simulink model "inverted_pendulum_simulink"  (R2023a)
settings: Solver=VariableStepAuto  StartTime=0.0  StopTime=10  RelTol=1e-3
values from neighbouring files (symbols this model uses):
  A = double(A)    [Inverted_pendulum_compute.m]
  B = double(B)    [Inverted_pendulum_compute.m]
  K = lqr(sys, Q, R)    [Inverted_pendulum_compute.m]
settings Model: Creator=belov  LastModifiedBy=belov

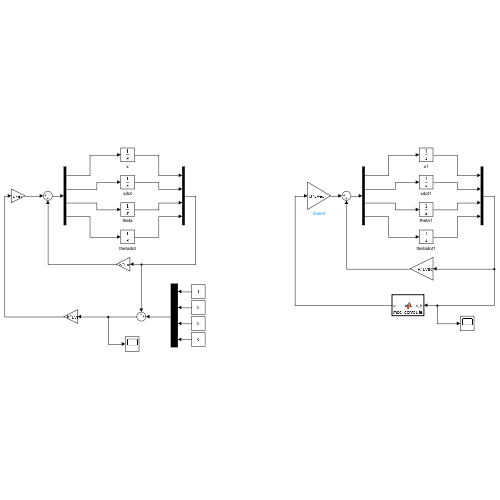
[thumbnail: Simulink's stored preview of the top-level diagram]
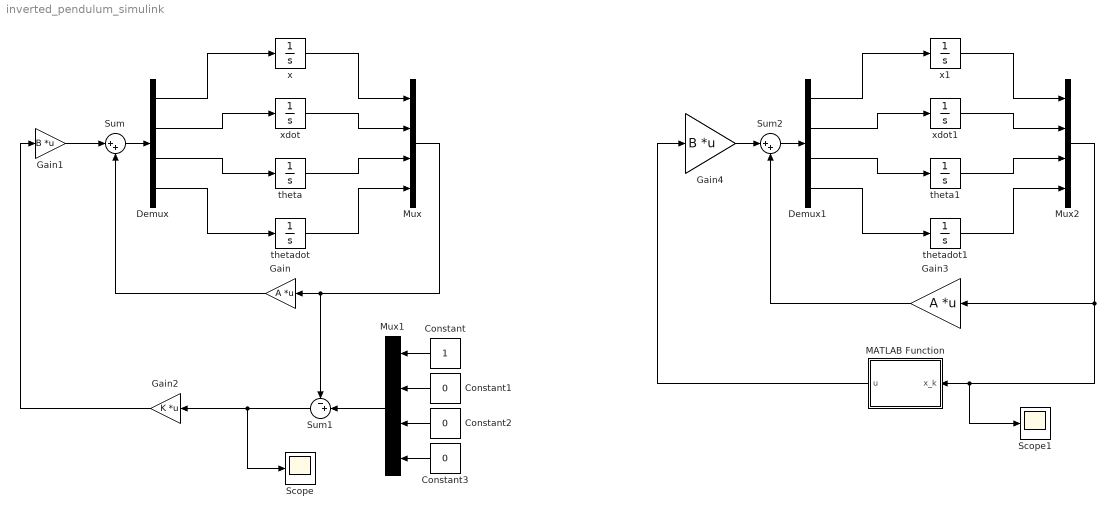
== system inverted_pendulum_simulink ==
  Constant : Constant
  Constant1 : Constant  Value=0
  Constant2 : Constant  Value=0
  Constant3 : Constant  Value=0
  Demux : Demux
  Demux1 : Demux
  Gain : Gain  Gain=A  Multiplication=Matrix(K*u) (u vector)
  Gain1 : Gain  Gain=B  Multiplication=Matrix(K*u) (u vector)
  Gain2 : Gain  Gain=K  Multiplication=Matrix(K*u) (u vector)
  Gain3 : Gain  Gain=A  Multiplication=Matrix(K*u) (u vector)
  Gain4 : Gain  Gain=B  Multiplication=Matrix(K*u) (u vector)
  MATLAB Function : MATLAB Function  TreatAsAtomicUnit=on  SystemSampleTime=0.01
  Mux : Mux
  Mux1 : Mux
  Mux2 : Mux
  Scope : Scope
  Scope1 : Scope
  Sum : Sum  Inputs=|++
  Sum1 : Sum  Inputs=-+|
  Sum2 : Sum  Inputs=|++
  theta : Integrator
  theta1 : Integrator
  thetadot : Integrator
  thetadot1 : Integrator
  x : Integrator
  x1 : Integrator  InitialCondition=1
  xdot : Integrator
  xdot1 : Integrator
  wires:
  Demux/1 -> x/1
  Demux/2 -> xdot/1
  Demux/3 -> theta/1
  Demux/4 -> thetadot/1
  x/1 -> Mux/1
  xdot/1 -> Mux/2
  theta/1 -> Mux/3
  thetadot/1 -> Mux/4
  Mux/1 -> Sum1/1, Gain/1
  Sum/1 -> Demux/1
  Gain/1 -> Sum/2
  Gain1/1 -> Sum/1
  Mux1/1 -> Sum1/2
  Constant/1 -> Mux1/1
  Constant1/1 -> Mux1/2
  Constant2/1 -> Mux1/3
  Constant3/1 -> Mux1/4
  Sum1/1 -> Scope/1, Gain2/1
  Gain2/1 -> Gain1/1
  Gain4/1 -> Sum2/1
  Gain3/1 -> Sum2/2
  Sum2/1 -> Demux1/1
  Mux2/1 -> Gain3/1, Scope1/1, MATLAB Function/1(x_k)
  thetadot1/1 -> Mux2/4
  theta1/1 -> Mux2/3
  xdot1/1 -> Mux2/2
  x1/1 -> Mux2/1
  Demux1/4 -> thetadot1/1
  Demux1/3 -> theta1/1
  Demux1/2 -> xdot1/1
  Demux1/1 -> x1/1
  MATLAB Function/1(u) -> Gain4/1

== matlab function inverted_pendulum_simulink/MATLAB Function ==
  data: x_k input; u output
function u = mpc_compute(x_k)

A = [ 1.0000    0.0100   -0.0002   -0.0000;
         0    1.0000   -0.0392   -0.0002;
         0         0    1.0010    0.0100;
         0         0    0.1962    1.0010;];
B = [ 0.0001;
    0.0200;
   -0.0001;
   -0.0286];
Q = diag([10, 1, 100, 1]);
R = diag(1);
N = 2;
n=size(A,1);
p=size(B,2);
M=[eye(n);zeros(N*n,n)];
C=zeros((N+1)*n,N*p);
tmp=eye(n);
for i=1:N
    rows =i*n+(1:n); 
    C(rows,:)=[tmp*B,C(rows-n, 1:end-p)];
    tmp= A*tmp;
    M(rows,:)=tmp;
end
% 定义Q_bar和R_bar
Q_bar = kron(eye(N),Q);
Q_bar = blkdiag(Q_bar,Q);
R_bar = kron(eye(N),R);
% 计算G, E, H
G = M'*Q_bar*M;
E = C'*Q_bar*M;
H = C'*Q_bar*C+R_bar;

U_k = zeros(N*p,1);
opts = optimoptions('quadprog','Algorithm','active-set');
U_k = quadprog(H, E * x_k, [], [], [], [], [], [], zeros(size(H, 1), 1), opts);
u = U_k(1, 1);
